simulink model "ques7_ref_model"  (R2021a)
settings: Solver=VariableStepAuto  StartTime=0.0  StopTime=10.0  RelTol=1e-3
settings Model: Creator=AVM  LastModifiedBy=AVM
settings DataIOCC: SaveOutput=off  SaveTime=off

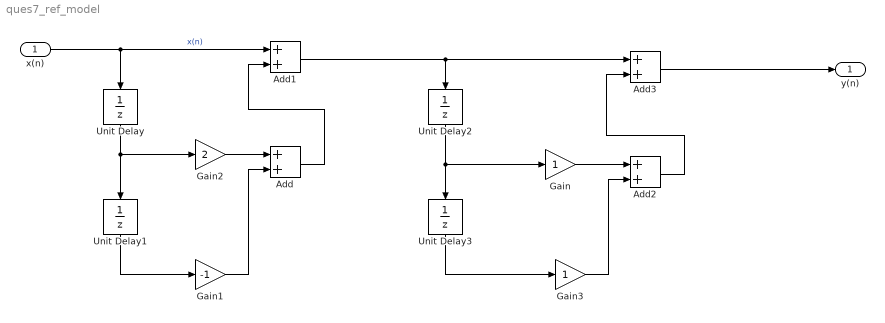
== system ques7_ref_model ==
  x(n) : Inport  OutDataTypeStr=double  PortDimensions=1  SampleTime=0
  Add{,1..3} (4 alike) : Sum
  Gain : Gain
  Gain1 : Gain  Gain=-1
  Gain2 : Gain  Gain=2
  Gain3 : Gain
  Unit Delay{,1..3} (4 alike) : UnitDelay  SampleTime=-1  HasFrameUpgradeWarning=on
  y(n) : Outport  OutDataTypeStr=double  PortDimensions=1  SampleTime=0
  wires:
  Add3/1 -> y(n)/1
  Add/1 -> Add1/2
  Unit Delay2/1 -> Gain/1, Unit Delay3/1
  Unit Delay/1 -> Unit Delay1/1, Gain2/1
  Add1/1 -> Unit Delay2/1, Add3/1
  x(n)/1 -> Add1/1, Unit Delay/1  "x(n)"
  Add2/1 -> Add3/2
  Gain1/1 -> Add/2
  Unit Delay3/1 -> Gain3/1
  Unit Delay1/1 -> Gain1/1
  Gain3/1 -> Add2/2
  Gain/1 -> Add2/1
  Gain2/1 -> Add/1
